simulink model "modelagem_2021a_1"  (R2021a)
settings: Solver=VariableStepAuto  StartTime=0.0  StopTime=3  FixedStep=10^-5  MaxStep=10^-4  RelTol=1e-3
StopFcn:
  | q = out.logsout{2}.Values;
  | wc = out.logsout{1}.Values;
  | figure(1)
  | plot(q.Time,q.Data)
  | 
  | hold off
  | figure(2)
  | plot(wc.Time,wc.Data)
  | legend("\omega_x","\omega_y","\omega_z")
  | ylabel("Velocidade Angular [rad/s]")
  | xlabel("Tempo [s]")
values from neighbouring files (symbols this model uses):
  b = 17.03*10^(-6)    (= 1.703e-05)    [modelagem_script.m]
  g = [0;0;-9.81]    [modelagem_script.m]
  Ic = [0.01008 -0.00309375 -0.00309375 ... (first row only)    [modelagem_script.m]
  Ic_inv = inv(Ic)    [modelagem_script.m]
  mc = 0.55    [modelagem_script.m]
  q00 = [cos(phi_u/2);e_u*sin(phi_u/2)]    [modelagem_script.m]
  rc = [0.0954545;0.0954545;0.0954545]    [modelagem_script.m]
  Tau = [0;0;0]    [modelagem_script.m]
  w00 = [0;0;0]    [modelagem_script.m]
libraries: vrlib x2
settings Model: Creator=guimi  LastModifiedBy=guimi
settings DebuggingCC: UnconnectedInputMsg=none  UnconnectedOutputMsg=none  UnconnectedLineMsg=none
settings ModelReferenceCC: EnableRefExpFcnMdlSchedulingChecks=off
settings RTWCC: Description=Generic Real-Time Target  DLArmComputeVersion=20.02.1

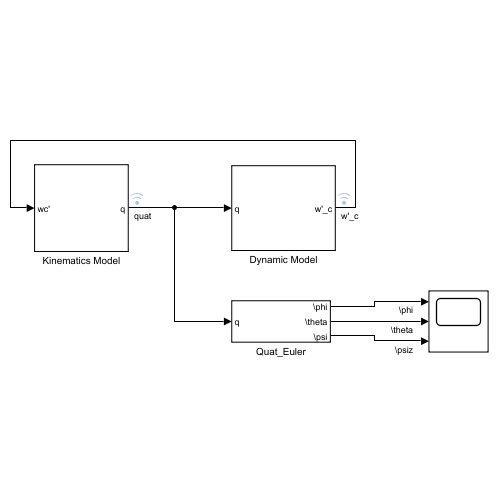
[thumbnail: Simulink's stored preview of the top-level diagram]
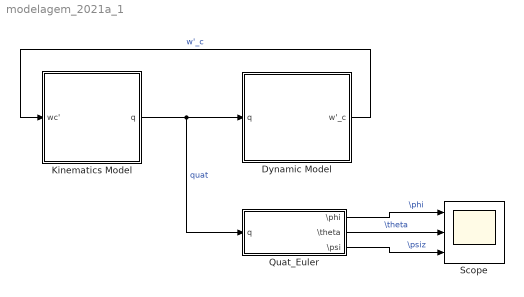
== system modelagem_2021a_1 ==
  Dynamic Model : Subsystem
  Kinematics Model : Subsystem
  Quat_Euler : Subsystem
  Scope : Scope  NumInputPorts=3
  wires:
  Kinematics Model/1(q) -> Quat_Euler/1(q), Dynamic Model/1(q)  "quat"
  Dynamic Model/1(w'_c) -> Kinematics Model/1(wc')  "w'_c"
  Quat_Euler/1(\phi) -> Scope/1  "\\phi"
  Quat_Euler/2(\theta) -> Scope/2  "\\theta"
  Quat_Euler/3(\psi) -> Scope/3  "\\psiz"

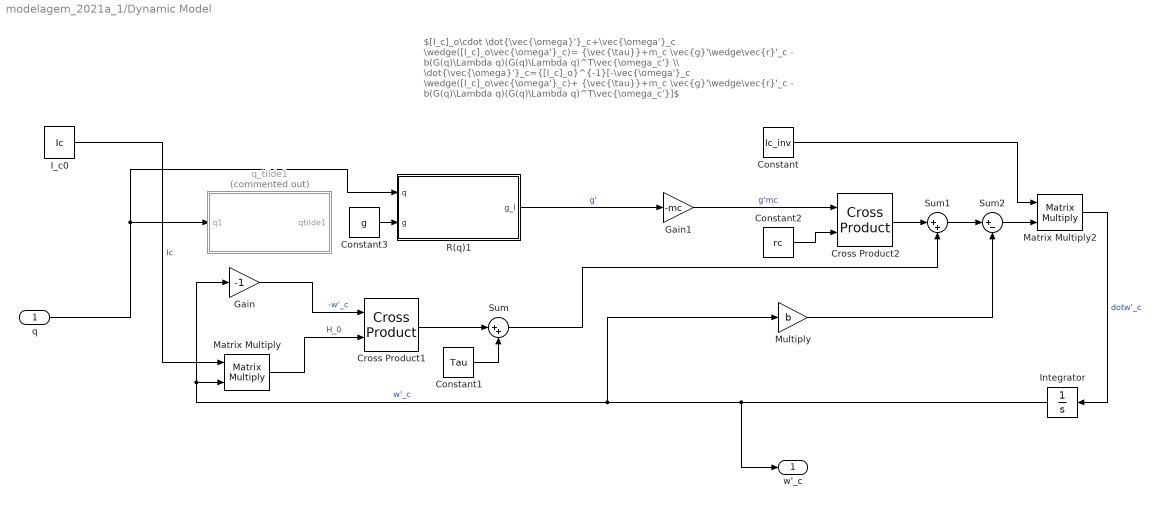
== system modelagem_2021a_1/Dynamic Model ==
  note: $[I_c]_o\cdot \dot{\vec{\omega}'}_c+\vec{\omega'}_c \wedge([I_c]_o\vec{\omega'}_c)= {\vec{\tau}}+m_c \vec{g}'\wedge\vec{r}'_c - b(G(q)\Lambda q)(G(q)\Lambda q)^T\vec{\omega_c'} \\ \dot{\vec{\omega}'}_c={[I_c]_o}^{-1}[-\vec{\omega'}_c \wedge([I_c]_o\vec{\omega'}_c)+ {\vec{\tau}}+m_c \vec{g}'\wedge\vec{r}'_c - b(G(q)\Lambda q)(G(q)\Lambda q)^T\vec{\omega_c'}]$
  q : Inport
  Constant : Constant  Value=Ic_inv
  Constant1 : Constant  Value=Tau
  Constant2 : Constant  Value=rc
  Constant3 : Constant  Value=g
  Cross Product1 : vrlib/Utilities/Cross Product
  Cross Product2 : vrlib/Utilities/Cross Product
  Gain : Gain  Gain=-1
  Gain1 : Gain  Gain=-mc
  I_c0 : Constant  Value=Ic
  Integrator : Integrator  InitialCondition=w00
  Matrix Multiply : Product  Multiplication=Matrix(*)
  Matrix Multiply2 : Product  Multiplication=Matrix(*)
  Multiply : Gain  Gain=b
  R(q)1 : MATLAB Function  TreatAsAtomicUnit=on
  Sum : Sum  Inputs=|++
  Sum1 : Sum  Inputs=|++
  Sum2 : Sum  Inputs=|+-
  q_tilde1 : Subsystem  Commented=on
  w'_c : Outport
  wires:
  I_c0/1 -> Matrix Multiply/1  "Ic"
  Integrator/1 -> Matrix Multiply/2, Gain/1, Multiply/1, w'_c/1  "w'_c"
  Matrix Multiply/1 -> Cross Product1/2  "H_0"
  Gain/1 -> Cross Product1/1  "-w'_c"
  Cross Product1/1 -> Sum/1
  Constant1/1 -> Sum/2
  q/1 -> R(q)1/1(q), q_tilde1/1(q1)
  Gain1/1 -> Cross Product2/1  "g'mc"
  Constant2/1 -> Cross Product2/2
  Sum/1 -> Sum1/2
  Sum1/1 -> Sum2/1
  Multiply/1 -> Sum2/2
  Sum2/1 -> Matrix Multiply2/2
  Constant/1 -> Matrix Multiply2/1
  Matrix Multiply2/1 -> Integrator/1  "dotw'_c"
  Cross Product2/1 -> Sum1/1
  R(q)1/1(g_l) -> Gain1/1  "g'"
  Constant3/1 -> R(q)1/2(g)

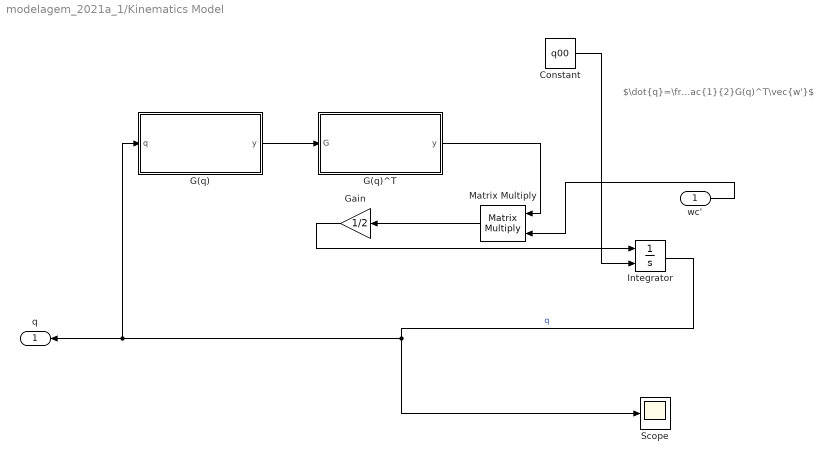
== system modelagem_2021a_1/Kinematics Model ==
  note: $\dot{q}=\frac{1}{2}G(q)^T\vec{w'}$
  wc' : Inport
  Constant : Constant  Value=q00
  G(q) : MATLAB Function  TreatAsAtomicUnit=on
  G(q)^T : MATLAB Function  TreatAsAtomicUnit=on
  Gain : Gain  Gain=1/2
  Integrator : Integrator  InitialConditionSource=external  InitialCondition=q00  UpperSaturationLimit=1  LowerSaturationLimit=-1
  Matrix Multiply : Product  Multiplication=Matrix(*)
  Scope : Scope
  q : Outport
  wires:
  G(q)/1(y) -> G(q)^T/1(G)
  wc'/1 -> Matrix Multiply/2
  G(q)^T/1(y) -> Matrix Multiply/1
  Integrator/1 -> Scope/1, G(q)/1(q), q/1  "q"
  Matrix Multiply/1 -> Gain/1
  Constant/1 -> Integrator/2
  Gain/1 -> Integrator/1

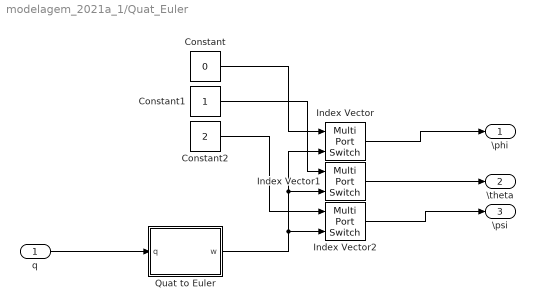
== system modelagem_2021a_1/Quat_Euler ==
  q : Inport
  Constant : Constant  Value=0
  Constant1 : Constant
  Constant2 : Constant  Value=2
  Index Vector : MultiPortSwitch  DataPortOrder=Zero-based contiguous  Inputs=1  zeroidx=on
  Index Vector1 : MultiPortSwitch  DataPortOrder=Zero-based contiguous  Inputs=1  zeroidx=on
  Index Vector2 : MultiPortSwitch  DataPortOrder=Zero-based contiguous  Inputs=1  zeroidx=on
  Quat to Euler : MATLAB Function  TreatAsAtomicUnit=on
  \phi : Outport
  \theta : Outport  Port=2
  \psi : Outport  Port=3
  wires:
  q/1 -> Quat to Euler/1(q)
  Quat to Euler/1(w) -> Index Vector/2, Index Vector1/2, Index Vector2/2
  Constant2/1 -> Index Vector2/1
  Constant1/1 -> Index Vector1/1
  Constant/1 -> Index Vector/1
  Index Vector/1 -> \phi/1
  Index Vector1/1 -> \theta/1
  Index Vector2/1 -> \psi/1

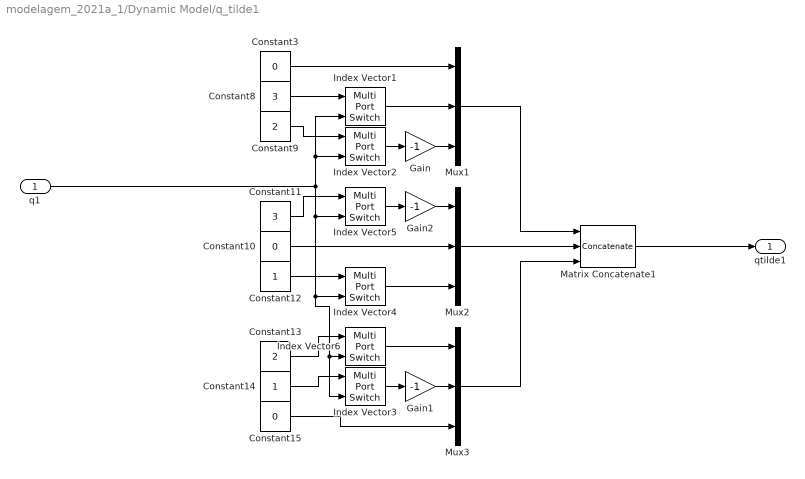
== system modelagem_2021a_1/Dynamic Model/q_tilde1 ==
  q1 : Inport
  Constant10 : Constant  Value=0
  Constant11 : Constant  Value=3
  Constant12 : Constant
  Constant13 : Constant  Value=2
  Constant14 : Constant
  Constant15 : Constant  Value=0
  Constant3 : Constant  Value=0
  Constant8 : Constant  Value=3
  Constant9 : Constant  Value=2
  Gain : Gain  Gain=-1
  Gain1 : Gain  Gain=-1
  Gain2 : Gain  Gain=-1
  Index Vector{1..6} (6 alike) : MultiPortSwitch  DataPortOrder=Zero-based contiguous  Inputs=1  zeroidx=on
  Matrix Concatenate1 : Concatenate  NumInputs=3  Mode=Multidimensional array  ConcatenateDimension=2
  Mux1 : Mux  Inputs=3
  Mux2 : Mux  Inputs=3
  Mux3 : Mux  Inputs=3
  qtilde1 : Outport
  wires:
  q1/1 -> Index Vector5/2, Index Vector3/2, Index Vector6/2, Index Vector4/2, Index Vector1/2, Index Vector2/2
  Constant3/1 -> Mux1/1
  Constant8/1 -> Index Vector1/1
  Index Vector1/1 -> Mux1/2
  Constant9/1 -> Index Vector2/1
  Index Vector2/1 -> Gain/1
  Gain/1 -> Mux1/3
  Index Vector4/1 -> Mux2/3
  Constant10/1 -> Mux2/2
  Index Vector5/1 -> Gain2/1
  Gain2/1 -> Mux2/1
  Constant11/1 -> Index Vector5/1
  Constant12/1 -> Index Vector4/1
  Index Vector6/1 -> Mux3/1
  Constant15/1 -> Mux3/3
  Constant13/1 -> Index Vector6/1
  Constant14/1 -> Index Vector3/1
  Index Vector3/1 -> Gain1/1
  Gain1/1 -> Mux3/2
  Mux2/1 -> Matrix Concatenate1/2
  Mux1/1 -> Matrix Concatenate1/1
  Mux3/1 -> Matrix Concatenate1/3
  Matrix Concatenate1/1 -> qtilde1/1

== matlab function modelagem_2021a_1/Quat_Euler/Quat to Euler ==
  data: q input; w output
function w = fcn(q)

    phi = atan2(q(4),q(1)) - atan2(-q(2),q(3));
    theta = acos((2*(q(1)^2+q(4)^2))-1);
    psi = atan2(q(4),q(1)) + atan2(-q(2),q(3));

w = [phi;theta;psi];

== matlab function modelagem_2021a_1/Kinematics Model/G(q) ==
  data: q input; y output
function y = fcn(q)
    y = [-q(2) q(1) q(4) -q(3); -q(3) -q(4) q(1) q(2); -q(4) q(3) -q(2) q(1)];  
end

== matlab function modelagem_2021a_1/Kinematics Model/G(q)^T ==
  data: G input; y output
function y = fcn(G)
    y = G.';  
end

== matlab function modelagem_2021a_1/Dynamic Model/R(q)1 ==
  data: q input; g_l output; g input
function g_l = fcn(q,g)
    I = eye(3);
    qi = [q(2);q(3);q(4)];
    qT = qi.';
    g_l = 2*dot(qi,g)*qi + q(1)^2*g + 2*q(1)*cross(g,qi) - dot(qi,qi)*g;
end
